simulink model "mVeh_tbm"  (R2020a)
settings: configuration reference "config_cnv" (kept outside this file)
undefined symbols (not defined in the file): Calib_pirelle_presSnr_x8, Calib_roadTriger_x6, Calib_tbm_brkBts_x8, Calib_tbm_ctr_x8, Calib_tbm_sensor_x4, Calib_tbm_strDistb_x8, Calib_tbm_supCtr_x8, CtrSet_tbm_enab_x8, FtIME_CAN_LINEoFF_ecuTbm_pd, Parm_tbmVeh_sig_max_numInvalid, Parm_tbmVeh_sig_tolerate_numInvalid, sigbuilder_block, SwCfg_cuTbm_simuCan
libraries: lib_canRx_msg_v2 x3, simulink x1, lib_decmp_Calib_tbm_brkPreTriger_x6 x1, lib_decmp_CtrSet_tbm_enab_x8 x1, libmf_bcu_spd_stsToValid x1, lib_decmp_Calib_tbm_sensor_x4 x1
settings Model: PauseTimes=30.8  Creator=jianjun.gao  LastModifiedBy=Administrator
settings ConfigSetRef: SourceName=config_cnv  SourceLocation=Base Workspace

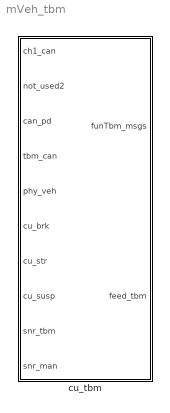
== system mVeh_tbm ==
  cu_tbm : Subsystem

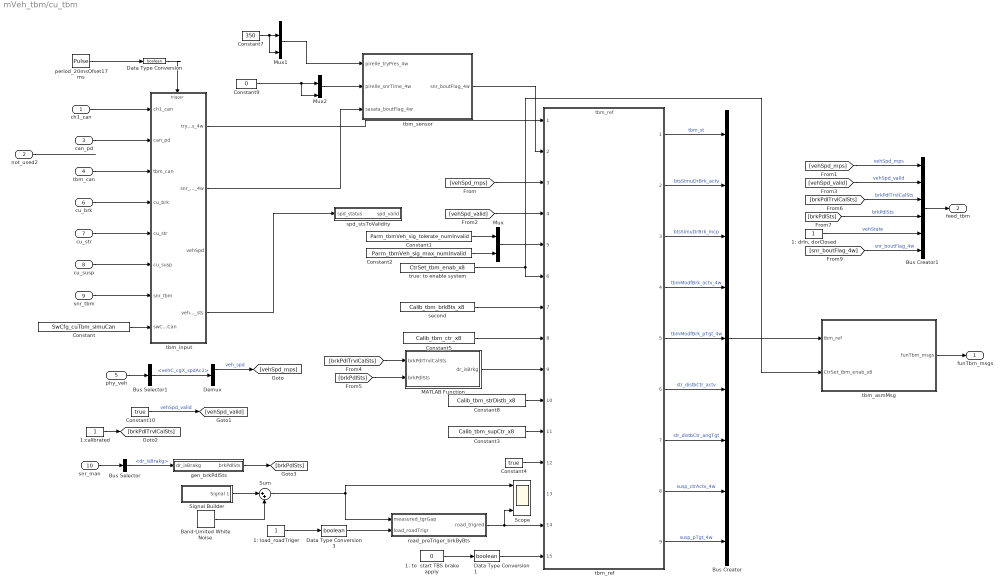
== system mVeh_tbm/cu_tbm ==
  ch1_can : Inport
  not_used2 : Inport  Port=2
  can_pd : Inport  Port=3
  tbm_can : Inport  Port=4
  phy_veh : Inport  Port=5
  cu_brk : Inport  Port=6
  cu_str : Inport  Port=7
  cu_susp : Inport  Port=8
  snr_tbm : Inport  Port=9
  snr_man : Inport  Port=10
  "1: drIn, dorClosed" : Constant  OutDataTypeStr=single  SampleTime=-1
  1: load_roadTriger : Constant  OutDataTypeStr=uint8  SampleTime=-1
  1: to  start TBS brake apply : Constant  Value=0  OutDataTypeStr=uint8  SampleTime=-1
  1:calibrated : Constant  OutDataTypeStr=uint8  SampleTime=-1
  Band-Limited White Noise : simulink/Sources/Band-Limited White Noise  Cov=[0.00000000001]  Ts=0.001  seed=[0]
  Bus Creator : BusCreator  Inputs=9
  Bus Creator1 : BusCreator  Inputs=6
  Bus Selector : BusSelector  OutputSignals=dr_isBrakg
  Bus Selector1 : BusSelector  OutputSignals=vehC_cgX_spdAc2
  Constant : Constant  Value=SwCfg_cuTbm_simuCan  OutDataTypeStr=boolean  SampleTime=-1
  Constant1 : Constant  Value=Parm_tbmVeh_sig_tolerate_numInvalid  OutDataTypeStr=int8  SampleTime=-1
  Constant10 : Constant  Value=true  OutDataTypeStr=boolean  SampleTime=-1
  Constant2 : Constant  Value=Parm_tbmVeh_sig_max_numInvalid  OutDataTypeStr=int8  SampleTime=-1
  Constant3 : Constant  Value=Calib_tbm_supCtr_x8  OutDataTypeStr=single  SampleTime=-1
  Constant4 : Constant  Value=true  OutDataTypeStr=boolean  SampleTime=-1
  Constant5 : Constant  Value=Calib_tbm_ctr_x8  OutDataTypeStr=single  SampleTime=-1
  Constant7 : Constant  Value=350  OutDataTypeStr=single  SampleTime=-1
  Constant8 : Constant  Value=Calib_tbm_strDistb_x8  OutDataTypeStr=single  SampleTime=-1
  Constant9 : Constant  Value=0  OutDataTypeStr=single  SampleTime=-1
  Data Type Conversion : DataTypeConversion  OutDataTypeStr=boolean  RndMeth=Nearest
  Data Type Conversion1 : DataTypeConversion  OutDataTypeStr=boolean  RndMeth=Nearest
  Data Type Conversion3 : DataTypeConversion  OutDataTypeStr=boolean  RndMeth=Nearest
  Demux : Demux  Outputs=2
  MATLAB Function : MATLAB Function  TreatAsAtomicUnit=on
  Mux : Mux  Inputs=2
  Mux1 : Mux
  Mux2 : Mux
  Scope : Scope  NumInputPorts=4
  Signal Builder : Subsystem  Tag=STV Subsys  LoadFcn=sigbuilder_block('load');  StartFcn=sigbuilder_block('start');  StopFcn=sigbuilder_block('stop');  ClipboardFcn=sigbuilder_block('clipboard');  mask(Sigbuilder block){tuvar=[0:10]}
      mask help: Simulink:masks:SigbuilderBlock_MD
      mask init:
      | if ~strcmp(get_param(bdroot(gcbh),'SimulationStatus'),'stopped') tuvar = sigbuilder_block('maskInit'); end
      settings: CopyFcn=sigbuilder_block('copy');  DeleteFcn=sigbuilder_block('delete');  ModelCloseFcn=sigbuilder_block('modelClose');  PreSaveFcn=sigbuilder_block('preSave');  PauseFcn=sigbuilder_block('pause');  ContinueFcn=sigbuilder_block('continue');  NameChangeFcn=sigbuilder_block('namechange');  OpenFcn=sigbuilder_block('open',[6 30 1428 680.25 ]);  CloseFcn=sigbuilder_block('close');
      mask Display: plot(0, 0, 100, 100,[2, 2, 32, 32, 2], [68, 8, 8, 68, 68],[32, 2], [38, 38], [32, 19, 2],[53, 60, 44], [32, 17, 17, 2],[16, 16, 31, 31]);txt = getActiveGroup(gcbh);text(2, 100, txt,'verticalAlignment', 'top');
  Sum : Sum  Inputs=|++
  gen_brkPdlSts : MATLAB Function  TreatAsAtomicUnit=on
  period_20msOfset17ms : DiscretePulseGenerator  PulseType=Time based  Period=0.02  PulseWidth=50  PhaseDelay=0.017
  road_preTriger_brkByBts : Subsystem
  second : Constant  Value=Calib_tbm_brkBts_x8  OutDataTypeStr=single  SampleTime=-1
  spd_stsToValidity : MATLAB Function  TreatAsAtomicUnit=on
  tbm_asmMsg : Subsystem
  tbm_input : Subsystem
  tbm_ref : ModelReference  ModelNameDialog=tbm_ref.slx  SimulationMode=Normal  ModelReferenceVersion=1.927
  tbm_sensor : Subsystem
  true: to enable system : Constant  Value=CtrSet_tbm_enab_x8  OutDataTypeStr=boolean  SampleTime=-1
  funTbm_msgs : Outport
  feed_tbm : Outport  Port=2
  wires:
  Mux2/1 -> tbm_sensor/2(pirelle_snrTime_4w)
  Constant9/1 -> Mux2/2, Mux2/4
  tbm_sensor/1(snr_boutFlag_4w) -> tbm_ref/2
  Mux1/1 -> tbm_sensor/1(pirelle_tryPres_4w)
  Constant7/1 -> Mux1/2, Mux1/4
  road_preTriger_brkByBts/1(road_trigred) -> tbm_ref/14, Scope/4
  Band-Limited White Noise/1 -> Sum/2
  Data Type Conversion3/1 -> road_preTriger_brkByBts/2(load_roadTrigr)
  1: load_roadTriger/1 -> Data Type Conversion3/1
  Signal Builder/1(Signal 1) -> Sum/1
  Sum/1 -> road_preTriger_brkByBts/1(measured_tgrGap), Scope/1
  [snr_boutFlag_4w] -> Bus Creator1/6  "snr_boutFlag_4w"
  "1: drIn, dorClosed"/1 -> Bus Creator1/5  "vehState"
  [brkPdlSts] -> Bus Creator1/4  "brkPdlSts"
  [brkPdlTrvlCalSts] -> Bus Creator1/3  "brkPdlTrvlCalSts"
  [brkPdlSts] -> MATLAB Function/2(brkPdlSts)
  MATLAB Function/1(dr_isBrkg) -> tbm_ref/9
  gen_brkPdlSts/1(brkPdlSts) -> [brkPdlSts]
  [brkPdlTrvlCalSts] -> MATLAB Function/1(brkPdlTrvlCalSts)
  1:calibrated/1 -> [brkPdlTrvlCalSts]
  [vehSpd_valid] -> Bus Creator1/2  "vehSpd_valid"
  [vehSpd_valid] -> tbm_ref/4
  Constant10/1 -> [vehSpd_valid]  "vehSpd_valid"
  [vehSpd_mps] -> Bus Creator1/1  "vehSpd_mps"
  [vehSpd_mps] -> tbm_ref/3
  Demux/1 -> [vehSpd_mps]  "veh_spd"
  Bus Creator1/1 -> feed_tbm/1
  Bus Selector1/1 -> Demux/1  "<vehC_cgX_spdAc2>"
  tbm_asmMsg/1(funTbm_msgs) -> funTbm_msgs/1
  tbm_ref/6 -> Bus Creator/6  "str_distbCtr_actv"
  tbm_ref/7 -> Bus Creator/7  "str_distbCtr_angTgt"
  Constant4/1 -> tbm_ref/12
  tbm_ref/9 -> Bus Creator/9  "susp_pTgt_4w"
  tbm_ref/8 -> Bus Creator/8  "susp_ctrActv_4w"
  Constant3/1 -> tbm_ref/11
  Constant8/1 -> tbm_ref/10
  tbm_ref/5 -> Bus Creator/5  "tbmModfBrk_pTgt_4w"
  tbm_ref/4 -> Bus Creator/4  "tbmModfBrk_actv_4w"
  Bus Selector/1 -> gen_brkPdlSts/1(dr_isBrakg)  "<dr_isBrakg>"
  Data Type Conversion1/1 -> tbm_ref/15
  second/1 -> tbm_ref/7
  snr_man/1 -> Bus Selector/1
  Bus Creator/1 -> tbm_asmMsg/1(tbm_ref)
  tbm_input/4(vehSpd_sts) -> spd_stsToValidity/1(spd_status)
  tbm_input/2(snr_boutFlag_4w) -> tbm_sensor/3(sasata_boutFlag_4w)
  tbm_input/1(tryPres_4w) -> tbm_ref/1
  Mux/1 -> tbm_ref/5
  1: to  start TBS brake apply/1 -> Data Type Conversion1/1
  true: to enable system/1 -> tbm_asmMsg/2(CtrSet_tbm_enab_x8), tbm_ref/6
  Constant5/1 -> tbm_ref/8
  Constant2/1 -> Mux/2
  Constant1/1 -> Mux/1
  Data Type Conversion/1 -> tbm_input/Trigger
  cu_brk/1 -> tbm_input/4(cu_brk)
  period_20msOfset17ms/1 -> Data Type Conversion/1
  Constant/1 -> tbm_input/8(swCfg_simuCan)
  tbm_ref/3 -> Bus Creator/3  "btsSimuDrBrk_mcp"
  tbm_ref/2 -> Bus Creator/2  "btsSimuDrBrk_actv"
  tbm_ref/1 -> Bus Creator/1  "tbm_st"
  tbm_can/1 -> tbm_input/3(tbm_can)
  can_pd/1 -> tbm_input/2(can_pd)
  not_used2/1 -> ?
  ch1_can/1 -> tbm_input/1(ch1_can)
  phy_veh/1 -> Bus Selector1/1
  cu_str/1 -> tbm_input/5(cu_str)
  cu_susp/1 -> tbm_input/6(cu_susp)
  snr_tbm/1 -> tbm_input/7(snr_tbm)

== system mVeh_tbm/cu_tbm/Signal Builder ==
  Demux : Demux  Tag=STV Demux  Outputs=1
      settings: DisplayOption=none
  FromWs : FromWorkspace  Tag=STV FromWs  VariableName=tuvar
      SigBuilderData=|
      | common.afterFinalStr = 'Extrapolate'
      | common.sampleTime = 0
      | dataSet.timeRange = [0 40]
      | dataSet.name = 'Group 1'
      | sbobj.Groups.Name = 'Group 1'
      | sbobj.Groups.Signals.Name = 'Signal 1'
      | sbobj.Groups.Signals.XData = [0 13 13 13.3 13.3 40]
      | sbobj.Groups.Signals.YData = [0.528 0.528 0.222 0.222 0.53 0.53]
      | sbobj.Groups.TimeRange = [0 40]
  Signal 1 : Outport  Tag=STV Outport
  wires:
  FromWs/1 -> Demux/1
  Demux/1 -> Signal 1/1

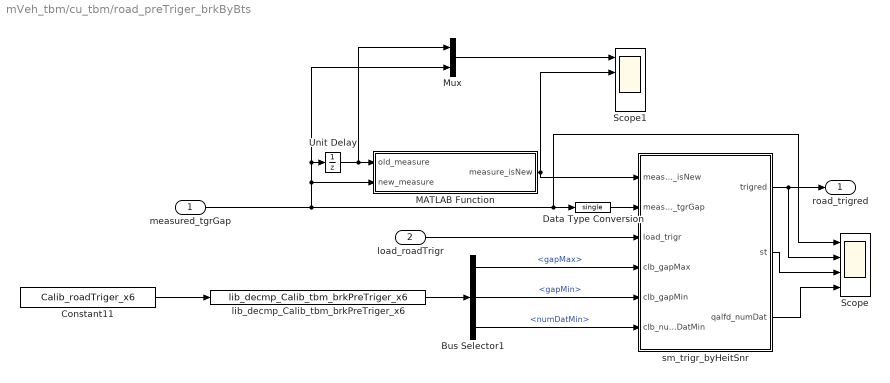
== system mVeh_tbm/cu_tbm/road_preTriger_brkByBts ==
  measured_tgrGap : Inport  OutDataTypeStr=double
  load_roadTrigr : Inport  Port=2  OutDataTypeStr=boolean
  Bus Selector1 : BusSelector  OutputSignals=gapMax,gapMin,numDatMin
  Constant11 : Constant  Value=Calib_roadTriger_x6  OutDataTypeStr=single  SampleTime=-1
  Data Type Conversion : DataTypeConversion  OutDataTypeStr=single
  MATLAB Function : MATLAB Function  TreatAsAtomicUnit=on
  Mux : Mux  Inputs=2
  Scope : Scope  NumInputPorts=4
  Scope1 : Scope  NumInputPorts=4
  Unit Delay : UnitDelay  SampleTime=-1  HasFrameUpgradeWarning=on
  lib_decmp_Calib_tbm_brkPreTriger_x6 : lib_decmp_Calib_tbm_brkPreTriger_x6/lib_decmp_Calib_tbm_brkPreTriger_x6  SystemSampleTime=-1  Latency=0  AutoFrameSizeCalculation=off
  sm_trigr_byHeitSnr : Stateflow chart  TreatAsAtomicUnit=on
  road_trigred : Outport
  wires:
  Data Type Conversion/1 -> sm_trigr_byHeitSnr/2(measured_tgrGap)
  Bus Selector1/3 -> sm_trigr_byHeitSnr/6(clb_numDatMin)  "<numDatMin>"
  Mux/1 -> Scope1/1
  sm_trigr_byHeitSnr/2(st) -> Scope/3
  sm_trigr_byHeitSnr/3(qalfd_numDat) -> Scope/4
  lib_decmp_Calib_tbm_brkPreTriger_x6/1 -> Bus Selector1/1
  Constant11/1 -> lib_decmp_Calib_tbm_brkPreTriger_x6/1
  sm_trigr_byHeitSnr/1(trigred) -> road_trigred/1, Scope/2
  load_roadTrigr/1 -> sm_trigr_byHeitSnr/3(load_trigr)
  measured_tgrGap/1 -> Data Type Conversion/1, Scope/1, MATLAB Function/2(new_measure), Unit Delay/1, Mux/2
  MATLAB Function/1(measure_isNew) -> Scope1/2, sm_trigr_byHeitSnr/1(measure_isNew)
  Unit Delay/1 -> MATLAB Function/1(old_measure), Mux/1
  Bus Selector1/1 -> sm_trigr_byHeitSnr/4(clb_gapMax)  "<gapMax>"
  Bus Selector1/2 -> sm_trigr_byHeitSnr/5(clb_gapMin)  "<gapMin>"

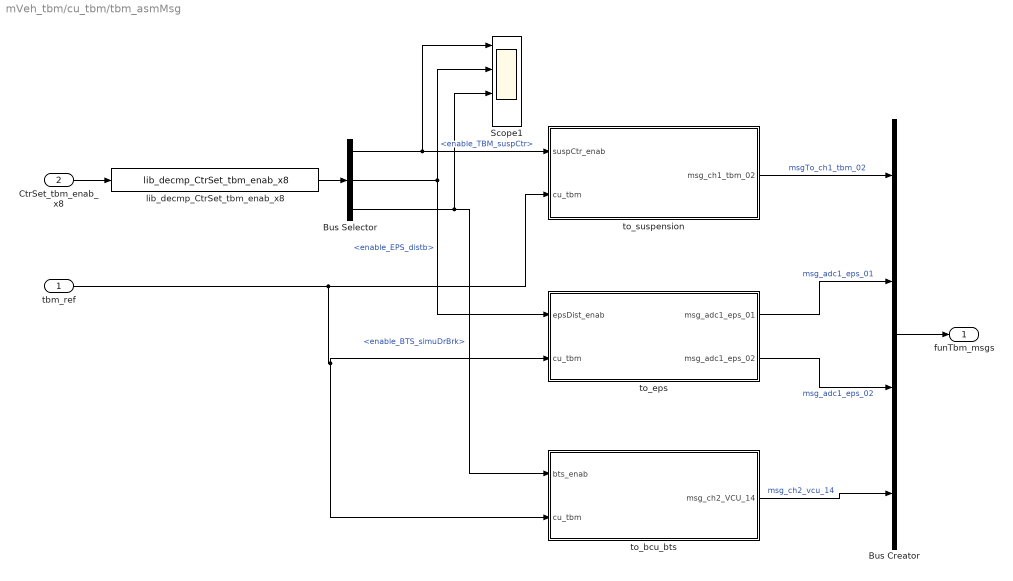
== system mVeh_tbm/cu_tbm/tbm_asmMsg ==
  tbm_ref : Inport
  CtrSet_tbm_enab_x8 : Inport  Port=2  OutDataTypeStr=boolean  PortDimensions=8
  Bus Creator : BusCreator  Inputs=4
  Bus Selector : BusSelector  OutputSignals=enable_TBM_suspCtr,enable_EPS_distb,enable_BTS_simuDrBrk
  Scope1 : Scope  NumInputPorts=4
  lib_decmp_CtrSet_tbm_enab_x8 : lib_decmp_CtrSet_tbm_enab_x8/lib_decmp_CtrSet_tbm_enab_x8  SystemSampleTime=-1  Latency=0  AutoFrameSizeCalculation=off
  to_bcu_bts : Subsystem
  to_eps : Subsystem
  to_suspension : Subsystem
  funTbm_msgs : Outport
  wires:
  Bus Creator/1 -> funTbm_msgs/1
  to_bcu_bts/1(msg_ch2_VCU_14) -> Bus Creator/4  "msg_ch2_vcu_14"
  to_eps/2(msg_adc1_eps_02) -> Bus Creator/3  "msg_adc1_eps_02"
  to_eps/1(msg_adc1_eps_01) -> Bus Creator/2  "msg_adc1_eps_01"
  to_suspension/1(msg_ch1_tbm_02) -> Bus Creator/1  "msgTo_ch1_tbm_02"
  Bus Selector/3 -> to_bcu_bts/1(bts_enab), Scope1/3  "<enable_BTS_simuDrBrk>"
  Bus Selector/2 -> to_eps/1(epsDist_enab), Scope1/2  "<enable_EPS_distb>"
  Bus Selector/1 -> to_suspension/1(suspCtr_enab), Scope1/1  "<enable_TBM_suspCtr>"
  lib_decmp_CtrSet_tbm_enab_x8/1 -> Bus Selector/1
  CtrSet_tbm_enab_x8/1 -> lib_decmp_CtrSet_tbm_enab_x8/1
  tbm_ref/1 -> to_suspension/2(cu_tbm), to_eps/2(cu_tbm), to_bcu_bts/2(cu_tbm)

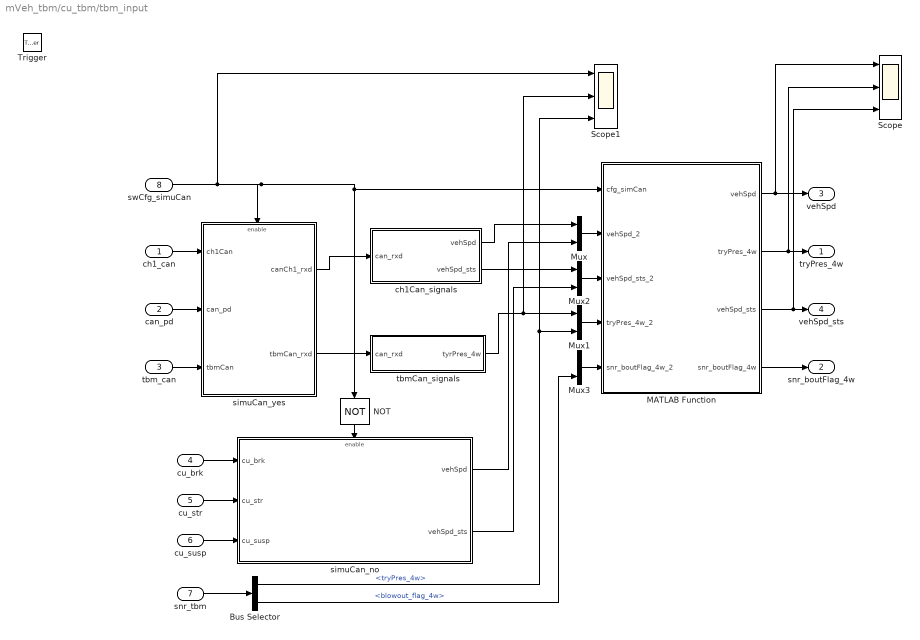
== system mVeh_tbm/cu_tbm/tbm_input ==
  ch1_can : Inport
  can_pd : Inport  Port=2
  tbm_can : Inport  Port=3
  cu_brk : Inport  Port=4
  cu_str : Inport  Port=5
  cu_susp : Inport  Port=6
  snr_tbm : Inport  Port=7
  swCfg_simuCan : Inport  Port=8
  Trigger : TriggerPort  TriggerType=either  VariantControl=Variant  PortDimensions=1
  Bus Selector : BusSelector  OutputSignals=tryPres_4w,blowout_flag_4w
  MATLAB Function : MATLAB Function  TreatAsAtomicUnit=on
  Mux{,1..3} (4 alike) : Mux  Inputs=2
  NOT : Logic  Operator=NOT  IconShape=distinctive  AllPortsSameDT=off  OutDataTypeStr=boolean
  Scope : Scope  NumInputPorts=3
  Scope1 : Scope  NumInputPorts=3
  ch1Can_signals : Subsystem
  simuCan_no : Subsystem
  simuCan_yes : Subsystem
  tbmCan_signals : Subsystem
  tryPres_4w : Outport
  snr_boutFlag_4w : Outport  Port=2
  vehSpd : Outport  Port=3
  vehSpd_sts : Outport  Port=4
  wires:
  MATLAB Function/4(snr_boutFlag_4w) -> snr_boutFlag_4w/1
  Mux3/1 -> MATLAB Function/5(snr_boutFlag_4w_2)
  Bus Selector/2 -> Mux3/2  "<blowout_flag_4w>"
  tbmCan_signals/1(tyrPres_4w) -> Mux1/1, Scope1/2
  simuCan_yes/2(tbmCan_rxd) -> tbmCan_signals/1(can_rxd)
  ch1Can_signals/2(vehSpd_sts) -> Mux2/1
  ch1Can_signals/1(vehSpd) -> Mux/1
  simuCan_yes/1(canCh1_rxd) -> ch1Can_signals/1(can_rxd)
  simuCan_no/2(vehSpd_sts) -> Mux2/2
  Mux2/1 -> MATLAB Function/3(vehSpd_sts_2)
  MATLAB Function/3(vehSpd_sts) -> Scope/3, vehSpd_sts/1
  MATLAB Function/2(tryPres_4w) -> Scope/2, tryPres_4w/1
  Mux1/1 -> MATLAB Function/4(tryPres_4w_2)
  MATLAB Function/1(vehSpd) -> Scope/1, vehSpd/1
  NOT/1 -> simuCan_no/Enable
  swCfg_simuCan/1 -> simuCan_yes/Enable, MATLAB Function/1(cfg_simCan), NOT/1, Scope1/1
  Mux/1 -> MATLAB Function/2(vehSpd_2)
  tbm_can/1 -> simuCan_yes/3(tbmCan)
  can_pd/1 -> simuCan_yes/2(can_pd)
  ch1_can/1 -> simuCan_yes/1(ch1Can)
  cu_susp/1 -> simuCan_no/3(cu_susp)
  cu_str/1 -> simuCan_no/2(cu_str)
  simuCan_no/1(vehSpd) -> Mux/2
  cu_brk/1 -> simuCan_no/1(cu_brk)
  snr_tbm/1 -> Bus Selector/1
  Bus Selector/1 -> Mux1/2, Scope1/3  "<tryPres_4w>"

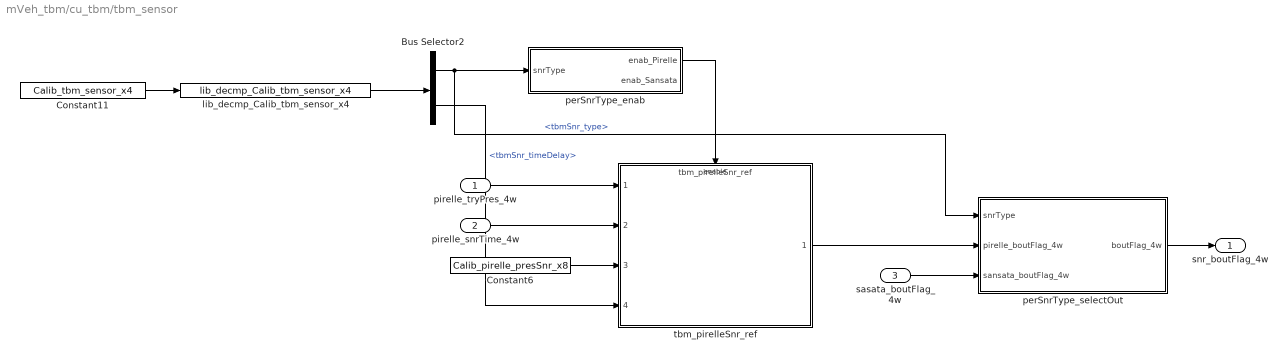
== system mVeh_tbm/cu_tbm/tbm_sensor ==
  pirelle_tryPres_4w : Inport  OutDataTypeStr=single  PortDimensions=4
  pirelle_snrTime_4w : Inport  Port=2  OutDataTypeStr=single  PortDimensions=4
  sasata_boutFlag_4w : Inport  Port=3  OutDataTypeStr=boolean  PortDimensions=4
  Bus Selector2 : BusSelector  OutputSignals=tbmSnr_type,tbmSnr_timeDelay
  Constant11 : Constant  Value=Calib_tbm_sensor_x4  SampleTime=-1
  Constant6 : Constant  Value=Calib_pirelle_presSnr_x8  OutDataTypeStr=single  SampleTime=-1
  lib_decmp_Calib_tbm_sensor_x4 : lib_decmp_Calib_tbm_sensor_x4/lib_decmp_Calib_tbm_sensor_x4  SystemSampleTime=-1  Latency=0  AutoFrameSizeCalculation=off
  perSnrType_enab : MATLAB Function  TreatAsAtomicUnit=on
  perSnrType_selectOut : MATLAB Function  TreatAsAtomicUnit=on
  tbm_pirelleSnr_ref : ModelReference  ModelNameDialog=tbm_pirelleSnr_ref.slx  SimulationMode=Normal  ModelReferenceVersion=1.851  EnablePortName=Enable  EnablePortStatesWhenEnabling=held
  snr_boutFlag_4w : Outport  OutDataTypeStr=boolean  PortDimensions=4
  wires:
  Bus Selector2/2 -> tbm_pirelleSnr_ref/4  "<tbmSnr_timeDelay>"
  pirelle_snrTime_4w/1 -> tbm_pirelleSnr_ref/2
  sasata_boutFlag_4w/1 -> perSnrType_selectOut/3(sansata_boutFlag_4w)
  tbm_pirelleSnr_ref/1 -> perSnrType_selectOut/2(pirelle_boutFlag_4w)
  perSnrType_selectOut/1(boutFlag_4w) -> snr_boutFlag_4w/1
  perSnrType_enab/1(enab_Pirelle) -> tbm_pirelleSnr_ref/Enable
  Bus Selector2/1 -> perSnrType_enab/1(snrType), perSnrType_selectOut/1(snrType)  "<tbmSnr_type>"
  Constant6/1 -> tbm_pirelleSnr_ref/3
  Constant11/1 -> lib_decmp_Calib_tbm_sensor_x4/1
  pirelle_tryPres_4w/1 -> tbm_pirelleSnr_ref/1
  lib_decmp_Calib_tbm_sensor_x4/1 -> Bus Selector2/1

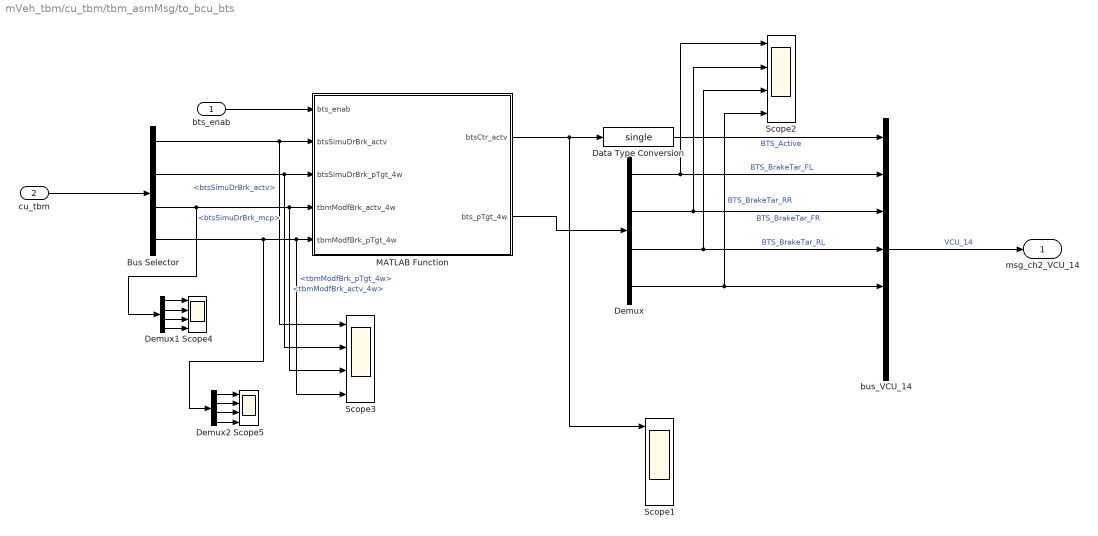
== system mVeh_tbm/cu_tbm/tbm_asmMsg/to_bcu_bts ==
  bts_enab : Inport
  cu_tbm : Inport  Port=2
  Bus Selector : BusSelector  OutputSignals=btsSimuDrBrk_actv,btsSimuDrBrk_mcp,tbmModfBrk_actv_4w,tbmModfBrk_pTgt_4w
  Data Type Conversion : DataTypeConversion  OutDataTypeStr=single  RndMeth=Nearest
  Demux : Demux
  Demux1 : Demux
  Demux2 : Demux
  MATLAB Function : MATLAB Function  TreatAsAtomicUnit=on
  Scope{1..5} (5 alike) : Scope  NumInputPorts=4
  bus_VCU_14 : BusCreator  Inputs=7
  msg_ch2_VCU_14 : Outport
  wires:
  Demux2/1 -> Scope5/1
  Demux2/2 -> Scope5/2
  Demux2/3 -> Scope5/3
  Demux2/4 -> Scope5/4
  Demux1/4 -> Scope4/4
  Demux1/3 -> Scope4/3
  Demux1/2 -> Scope4/2
  Demux1/1 -> Scope4/1
  MATLAB Function/2(bts_pTgt_4w) -> Demux/1
  Bus Selector/2 -> MATLAB Function/3(btsSimuDrBrk_pTgt_4w), Scope3/2  "<btsSimuDrBrk_mcp>"
  Bus Selector/4 -> MATLAB Function/5(tbmModfBrk_pTgt_4w), Scope3/4, Demux2/1  "<tbmModfBrk_pTgt_4w>"
  Bus Selector/3 -> MATLAB Function/4(tbmModfBrk_actv_4w), Scope3/3, Demux1/1  "<tbmModfBrk_actv_4w>"
  MATLAB Function/1(btsCtr_actv) -> Scope1/1, Data Type Conversion/1
  Bus Selector/1 -> MATLAB Function/2(btsSimuDrBrk_actv), Scope3/1  "<btsSimuDrBrk_actv>"
  Demux/4 -> bus_VCU_14/5, Scope2/4  "BTS_BrakeTar_RR"
  Demux/2 -> bus_VCU_14/3, Scope2/2  "BTS_BrakeTar_FR"
  bus_VCU_14/1 -> msg_ch2_VCU_14/1  "VCU_14"
  Data Type Conversion/1 -> bus_VCU_14/1  "BTS_Active"
  Demux/3 -> bus_VCU_14/4, Scope2/3  "BTS_BrakeTar_RL"
  Demux/1 -> bus_VCU_14/2, Scope2/1  "BTS_BrakeTar_FL"
  ? -> bus_VCU_14/7  "VCU_14_MsgCntr"
  ? -> bus_VCU_14/6  "VCU_14_CRC"
  cu_tbm/1 -> Bus Selector/1
  bts_enab/1 -> MATLAB Function/1(bts_enab)

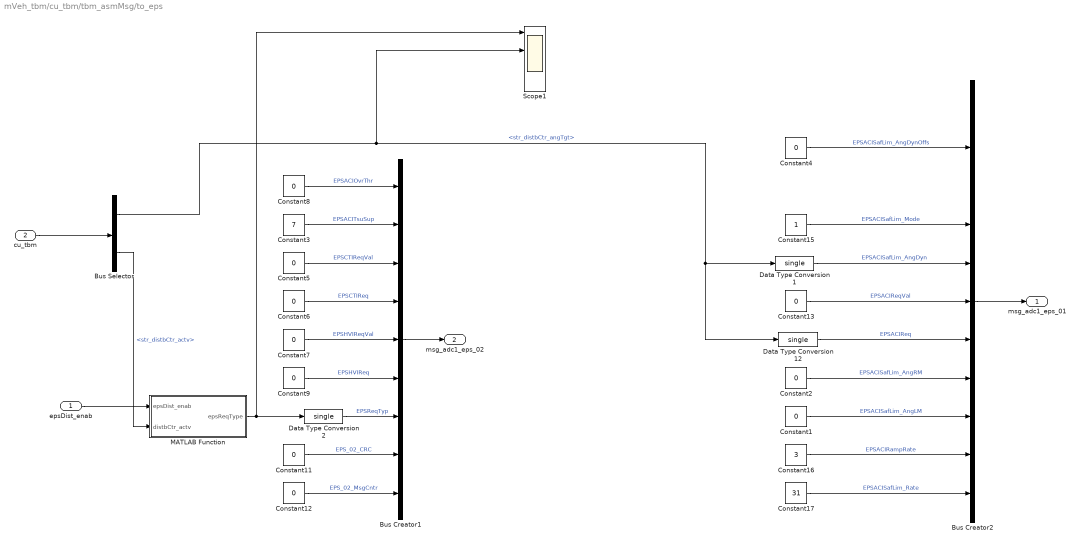
== system mVeh_tbm/cu_tbm/tbm_asmMsg/to_eps ==
  epsDist_enab : Inport
  cu_tbm : Inport  Port=2
  Bus Creator1 : BusCreator  Inputs=9
  Bus Creator2 : BusCreator  Inputs=11
  Bus Selector : BusSelector  OutputSignals=str_distbCtr_angTgt,str_distbCtr_actv
  Constant{1..2,4..9,11..13} (11 alike) : Constant  Value=0  OutDataTypeStr=single
  Constant15 : Constant  OutDataTypeStr=single
  Constant16 : Constant  Value=3  OutDataTypeStr=single
  Constant17 : Constant  Value=31  OutDataTypeStr=single
  Constant3 : Constant  Value=7  OutDataTypeStr=single
  Data Type Conversion1 : DataTypeConversion  OutDataTypeStr=single  RndMeth=Nearest
  Data Type Conversion12 : DataTypeConversion  OutDataTypeStr=single  RndMeth=Nearest
  Data Type Conversion2 : DataTypeConversion  OutDataTypeStr=single  RndMeth=Nearest
  MATLAB Function : MATLAB Function  TreatAsAtomicUnit=on
  Scope1 : Scope  NumInputPorts=4
  msg_adc1_eps_01 : Outport
  msg_adc1_eps_02 : Outport  Port=2
  wires:
  Data Type Conversion2/1 -> Bus Creator1/7  "EPSReqTyp"
  epsDist_enab/1 -> MATLAB Function/1(epsDist_enab)
  Bus Selector/2 -> MATLAB Function/2(distbCtr_actv)  "<str_distbCtr_actv>"
  cu_tbm/1 -> Bus Selector/1
  Constant15/1 -> Bus Creator2/4  "EPSACISafLim_Mode"
  Constant4/1 -> Bus Creator2/2  "EPSACISafLim_AngDynOffs"
  Constant5/1 -> Bus Creator1/3  "EPSCTIReqVal"
  Bus Creator1/1 -> msg_adc1_eps_02/1
  Constant8/1 -> Bus Creator1/1  "EPSACIOvrThr"
  Constant3/1 -> Bus Creator1/2  "EPSACITsuSup"
  Constant16/1 -> Bus Creator2/10  "EPSACIRampRate"
  Constant13/1 -> Bus Creator2/6  "EPSACIReqVal"
  Data Type Conversion12/1 -> Bus Creator2/7  "EPSACIReq"
  Constant6/1 -> Bus Creator1/4  "EPSCTIReq"
  Constant7/1 -> Bus Creator1/5  "EPSHVIReqVal"
  Bus Creator2/1 -> msg_adc1_eps_01/1
  Constant1/1 -> Bus Creator2/9  "EPSACISafLim_AngLM"
  Constant12/1 -> Bus Creator1/9  "EPS_02_MsgCntr"
  Data Type Conversion1/1 -> Bus Creator2/5  "EPSACISafLim_AngDyn"
  Constant17/1 -> Bus Creator2/11  "EPSACISafLim_Rate"
  MATLAB Function/1(epsReqType) -> Data Type Conversion2/1, Scope1/1
  Constant2/1 -> Bus Creator2/8  "EPSACISafLim_AngRM"
  ? -> Bus Creator2/1  "EPS_01_CRC"
  Constant11/1 -> Bus Creator1/8  "EPS_02_CRC"
  Constant9/1 -> Bus Creator1/6  "EPSHVIReq"
  Bus Selector/1 -> Data Type Conversion1/1, Data Type Conversion12/1, Scope1/2  "<str_distbCtr_angTgt>"
  ? -> Bus Creator2/3  "EPS_01_MsgCntr"

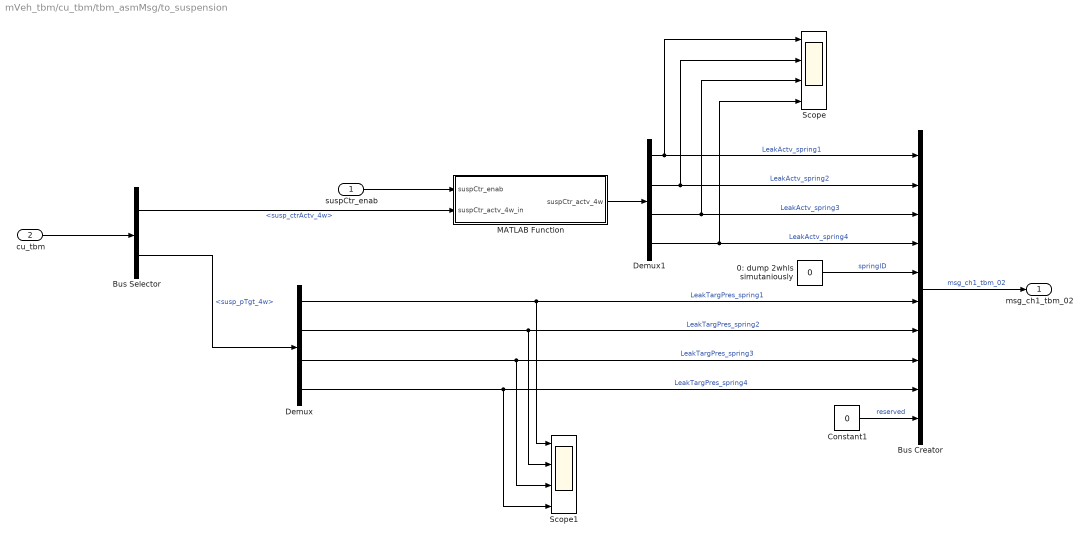
== system mVeh_tbm/cu_tbm/tbm_asmMsg/to_suspension ==
  suspCtr_enab : Inport
  cu_tbm : Inport  Port=2
  0: dump 2whls simutaniously : Constant  Value=0  OutDataTypeStr=single
  Bus Creator : BusCreator  Inputs=10
  Bus Selector : BusSelector  OutputSignals=susp_ctrActv_4w,susp_pTgt_4w
  Constant1 : Constant  Value=0  OutDataTypeStr=single
  Demux : Demux
  Demux1 : Demux
  MATLAB Function : MATLAB Function  TreatAsAtomicUnit=on
  Scope : Scope  NumInputPorts=4
  Scope1 : Scope  NumInputPorts=4
  msg_ch1_tbm_02 : Outport
  wires:
  suspCtr_enab/1 -> MATLAB Function/1(suspCtr_enab)
  MATLAB Function/1(suspCtr_actv_4w) -> Demux1/1
  Bus Selector/1 -> MATLAB Function/2(suspCtr_actv_4w_in)  "<susp_ctrActv_4w>"
  Bus Selector/2 -> Demux/1  "<susp_pTgt_4w>"
  Bus Creator/1 -> msg_ch1_tbm_02/1  "msg_ch1_tbm_02"
  Demux/1 -> Bus Creator/6, Scope1/1  "LeakTargPres_spring1"
  Demux1/3 -> Bus Creator/3, Scope/3  "LeakActv_spring3"
  Demux1/2 -> Bus Creator/2, Scope/2  "LeakActv_spring2"
  Constant1/1 -> Bus Creator/10  "reserved"
  Demux1/1 -> Bus Creator/1, Scope/1  "LeakActv_spring1"
  Demux/4 -> Bus Creator/9, Scope1/4  "LeakTargPres_spring4"
  Demux/3 -> Bus Creator/8, Scope1/3  "LeakTargPres_spring3"
  Demux/2 -> Bus Creator/7, Scope1/2  "LeakTargPres_spring2"
  Demux1/4 -> Bus Creator/4, Scope/4  "LeakActv_spring4"
  0: dump 2whls simutaniously/1 -> Bus Creator/5  "springID"
  cu_tbm/1 -> Bus Selector/1

== system mVeh_tbm/cu_tbm/tbm_input/ch1Can_signals ==
  can_rxd : Inport
  Bus Selector1 : BusSelector  OutputSignals=BCU_04_rxd
  Bus Selector2 : BusSelector  OutputSignals=BCU_04.VehSpd,BCU_04.VehSpdSts
  vehSpd : Outport
  vehSpd_sts : Outport  Port=2
  wires:
  Bus Selector2/2 -> vehSpd_sts/1  "<VehSpdSts>"
  Bus Selector2/1 -> vehSpd/1  "<VehSpd>"
  Bus Selector1/1 -> Bus Selector2/1  "<BCU_04_rxd>"
  can_rxd/1 -> Bus Selector1/1

== system mVeh_tbm/cu_tbm/tbm_input/simuCan_no ==
  cu_brk : Inport
  cu_str : Inport  Port=2
  cu_susp : Inport  Port=3
  Enable : EnablePort
  Bus Selector1 : BusSelector  OutputSignals=vehSpd,vehSpd_valid
  libmf_spd_validToSts : libmf_bcu_spd_stsToValid/libmf_spd_validToSts  SystemSampleTime=-1  Latency=0  AutoFrameSizeCalculation=off
  vehSpd : Outport
  vehSpd_sts : Outport  Port=2
  wires:
  libmf_spd_validToSts/1 -> vehSpd_sts/1
  Bus Selector1/2 -> libmf_spd_validToSts/1  "<vehSpd_valid>"
  cu_brk/1 -> Bus Selector1/1
  Bus Selector1/1 -> vehSpd/1  "<vehSpd>"

== system mVeh_tbm/cu_tbm/tbm_input/simuCan_yes ==
  ch1Can : Inport
  can_pd : Inport  Port=2
  tbmCan : Inport  Port=3
  Enable : EnablePort
  ch1Can_rx : Subsystem
  tbmCan_rx : Subsystem
  canCh1_rxd : Outport
  tbmCan_rxd : Outport  Port=2
  wires:
  tbmCan_rx/1(can_rxd) -> tbmCan_rxd/1
  tbmCan/1 -> tbmCan_rx/1(can)
  ch1Can_rx/1(can_rxd) -> canCh1_rxd/1
  ch1Can/1 -> ch1Can_rx/1(can)

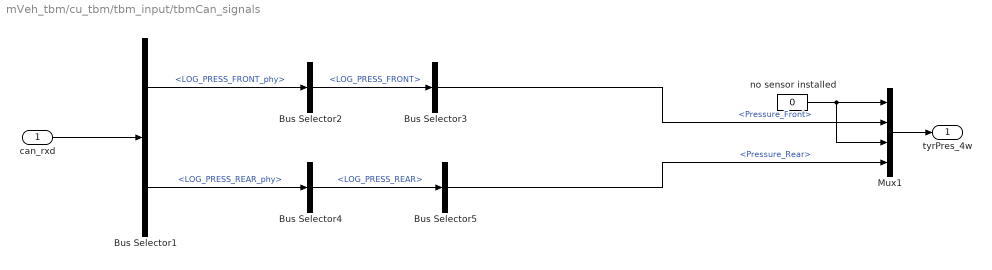
== system mVeh_tbm/cu_tbm/tbm_input/tbmCan_signals ==
  can_rxd : Inport
  Bus Selector1 : BusSelector  OutputSignals=LOG_PRESS_FRONT_phy,LOG_PRESS_REAR_phy
  Bus Selector2 : BusSelector  OutputSignals=LOG_PRESS_FRONT
  Bus Selector3 : BusSelector  OutputSignals=Pressure_Front
  Bus Selector4 : BusSelector  OutputSignals=LOG_PRESS_REAR
  Bus Selector5 : BusSelector  OutputSignals=Pressure_Rear
  Mux1 : Mux
  no sensor installed : Constant  Value=0  OutDataTypeStr=single  SampleTime=-1
  tyrPres_4w : Outport
  wires:
  no sensor installed/1 -> Mux1/1, Mux1/3
  Mux1/1 -> tyrPres_4w/1
  Bus Selector4/1 -> Bus Selector5/1  "<LOG_PRESS_REAR>"
  Bus Selector5/1 -> Mux1/4  "<Pressure_Rear>"
  Bus Selector3/1 -> Mux1/2  "<Pressure_Front>"
  Bus Selector1/2 -> Bus Selector4/1  "<LOG_PRESS_REAR_phy>"
  can_rxd/1 -> Bus Selector1/1
  Bus Selector1/1 -> Bus Selector2/1  "<LOG_PRESS_FRONT_phy>"
  Bus Selector2/1 -> Bus Selector3/1  "<LOG_PRESS_FRONT>"

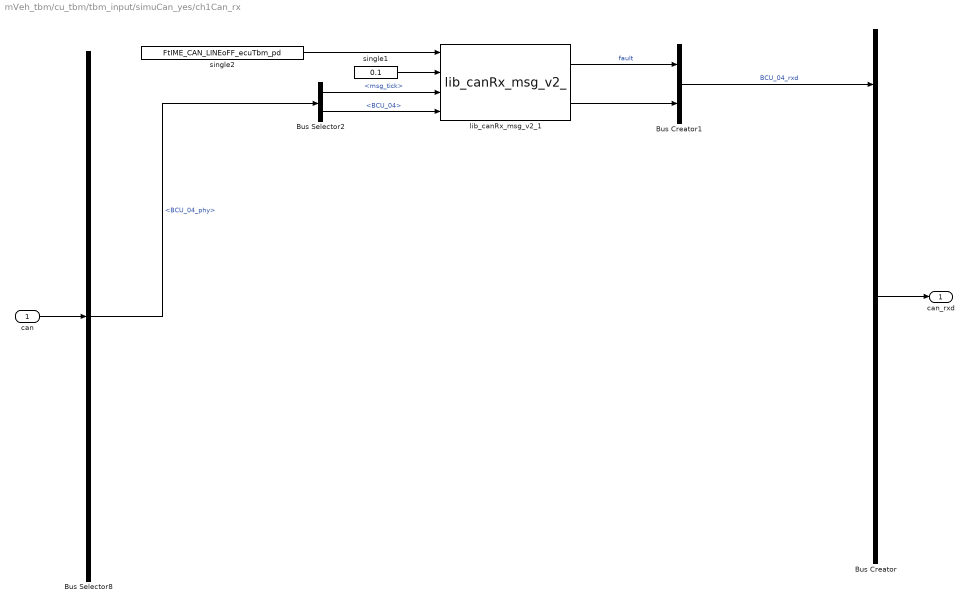
== system mVeh_tbm/cu_tbm/tbm_input/simuCan_yes/ch1Can_rx ==
  can : Inport
  Bus Creator : BusCreator  Inputs=5
  Bus Creator1 : BusCreator  Inputs=2
  Bus Selector2 : BusSelector  OutputSignals=msg_tick,BCU_04
  Bus Selector8 : BusSelector  OutputSignals=bcu.BCU_04_phy
  lib_canRx_msg_v2_1 : lib_canRx_msg_v2/lib_canRx_msg_v2_  SystemSampleTime=-1  Latency=0  AutoFrameSizeCalculation=off
  single1 : Constant  Value=0.1  OutDataTypeStr=single
  single2 : Constant  Value=FtIME_CAN_LINEoFF_ecuTbm_pd  OutDataTypeStr=single
  can_rxd : Outport  VectorParamsAs1DForOutWhenUnconnected=off
  wires:
  Bus Selector2/2 -> lib_canRx_msg_v2_1/4  "<BCU_04>"
  lib_canRx_msg_v2_1/1 -> Bus Creator1/1  "fault"
  Bus Selector2/1 -> lib_canRx_msg_v2_1/3  "<msg_tick>"
  single1/1 -> lib_canRx_msg_v2_1/2
  lib_canRx_msg_v2_1/2 -> Bus Creator1/2
  Bus Creator1/1 -> Bus Creator/1  "BCU_04_rxd"
  single2/1 -> lib_canRx_msg_v2_1/1
  can/1 -> Bus Selector8/1
  Bus Selector8/1 -> Bus Selector2/1  "<BCU_04_phy>"
  Bus Creator/1 -> can_rxd/1

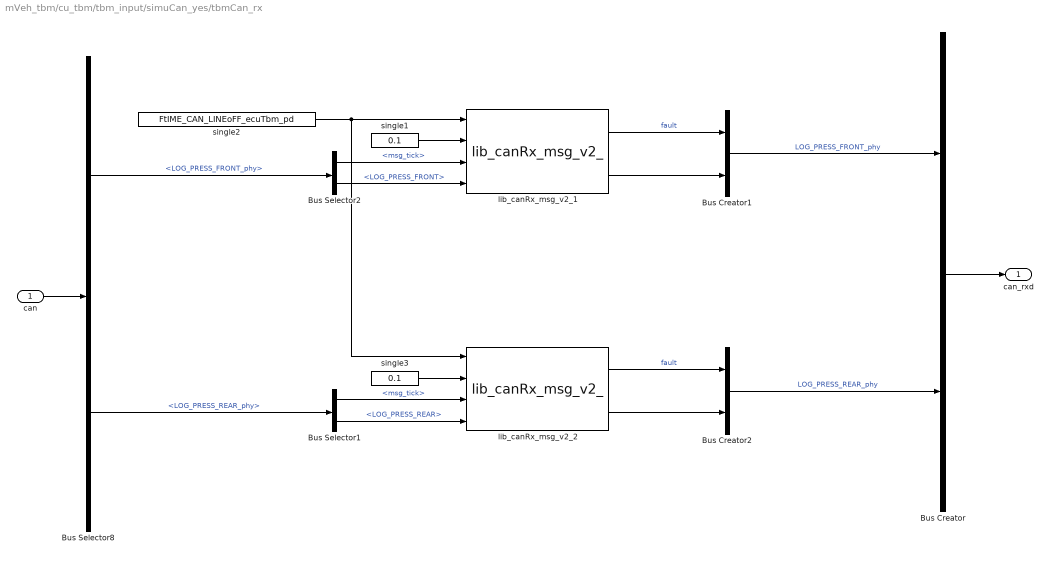
== system mVeh_tbm/cu_tbm/tbm_input/simuCan_yes/tbmCan_rx ==
  can : Inport
  Bus Creator : BusCreator  Inputs=2
  Bus Creator1 : BusCreator  Inputs=2
  Bus Creator2 : BusCreator  Inputs=2
  Bus Selector1 : BusSelector  OutputSignals=msg_tick,LOG_PRESS_REAR
  Bus Selector2 : BusSelector  OutputSignals=msg_tick,LOG_PRESS_FRONT
  Bus Selector8 : BusSelector  OutputSignals=tbm_pSnr.LOG_PRESS_FRONT_phy,tbm_pSnr.LOG_PRESS_REAR_phy
  lib_canRx_msg_v2_1 : lib_canRx_msg_v2/lib_canRx_msg_v2_  SystemSampleTime=-1  Latency=0  AutoFrameSizeCalculation=off
  lib_canRx_msg_v2_2 : lib_canRx_msg_v2/lib_canRx_msg_v2_  SystemSampleTime=-1  Latency=0  AutoFrameSizeCalculation=off
  single1 : Constant  Value=0.1  OutDataTypeStr=single
  single2 : Constant  Value=FtIME_CAN_LINEoFF_ecuTbm_pd  OutDataTypeStr=single
  single3 : Constant  Value=0.1  OutDataTypeStr=single
  can_rxd : Outport  VectorParamsAs1DForOutWhenUnconnected=off
  wires:
  Bus Selector8/2 -> Bus Selector1/1  "<LOG_PRESS_REAR_phy>"
  lib_canRx_msg_v2_2/1 -> Bus Creator2/1  "fault"
  lib_canRx_msg_v2_2/2 -> Bus Creator2/2
  single2/1 -> lib_canRx_msg_v2_1/1, lib_canRx_msg_v2_2/1
  Bus Selector1/2 -> lib_canRx_msg_v2_2/4  "<LOG_PRESS_REAR>"
  Bus Creator2/1 -> Bus Creator/2  "LOG_PRESS_REAR_phy"
  single3/1 -> lib_canRx_msg_v2_2/2
  Bus Selector1/1 -> lib_canRx_msg_v2_2/3  "<msg_tick>"
  Bus Creator/1 -> can_rxd/1
  Bus Selector8/1 -> Bus Selector2/1  "<LOG_PRESS_FRONT_phy>"
  can/1 -> Bus Selector8/1
  Bus Creator1/1 -> Bus Creator/1  "LOG_PRESS_FRONT_phy"
  lib_canRx_msg_v2_1/2 -> Bus Creator1/2
  single1/1 -> lib_canRx_msg_v2_1/2
  Bus Selector2/1 -> lib_canRx_msg_v2_1/3  "<msg_tick>"
  lib_canRx_msg_v2_1/1 -> Bus Creator1/1  "fault"
  Bus Selector2/2 -> lib_canRx_msg_v2_1/4  "<LOG_PRESS_FRONT>"

== matlab function mVeh_tbm/cu_tbm/road_preTriger_brkByBts/MATLAB Function ==
  data: old_measure input double; measure_isNew output boolean; new_measure input double
function measure_isNew = fcn(old_measure, new_measure)

measure_isNew = false;

if old_measure ~= new_measure
    measure_isNew = true;
end

== stateflow chart mVeh_tbm/cu_tbm/road_preTriger_brkByBts/sm_trigr_byHeitSnr ==
  state trigred
    en:
    st = 3;    trigred = true;
  state disregard
    en:
    st = 0;    trigred = false;
  state trigring
    en:
    st = 2;    trigred = false;
    state qualifed
      en:
      qalfd_numDat = qalfd_numDat +1;
    state unqualifed
      en:
      qalfd_numDat = qalfd_numDat -1;
    qualifed -> (junction 32)
    (junction 19) -> qualifed [order 1] : [      (measured_tgrGap < clb_gapMax) ...
        |   && (measured_tgrGap > clb_gapMin) ]
    (junction 32) -> (junction 19) : [measure_isNew]
    unqualifed -> (junction 32)
    (junction 19) -> unqualifed [order 2]
  state watch_for_trigr
    en:
    st = 1;    trigred = false;    qalfd_numDat = 0;
  (default) -> disregard
  trigred -> disregard : after(5, sec)
  trigring -> trigred [order 1] : [qalfd_numDat > clb_numDatMin ]
  disregard -> watch_for_trigr : [ load_trigr ]
  watch_for_trigr -> disregard [order 2] : [ ~load_trigr ]
  watch_for_trigr -> (junction 32) [order 1]
  trigring -> watch_for_trigr [order 2] : [qalfd_numDat <= 0 ]
  data: measure_isNew input boolean; measured_tgrGap input single size=1; load_trigr input boolean; clb_gapMax input single size=1; clb_gapMin input single size=1; trigred output boolean; clb_numDatMin input uint8 size=1; st output uint8; qalfd_numDat output uint8 size=1

== matlab function mVeh_tbm/cu_tbm/tbm_sensor/perSnrType_enab ==
  data: snrType input Enum: Enum_tbm_snrType; enab_Pirelle output boolean; enab_Sansata output boolean
function [enab_Pirelle,enab_Sansata] = fcn(snrType)

enab_Pirelle = false;
enab_Sansata = false;

switch snrType
    case Enum_tbm_snrType.Pirelle
        enab_Pirelle = true;
    case Enum_tbm_snrType.Sansata  
        enab_Sansata = true;
    
end

== matlab function mVeh_tbm/cu_tbm/tbm_sensor/perSnrType_selectOut ==
  data: snrType input Enum: Enum_tbm_snrType; boutFlag_4w output boolean size=4; pirelle_boutFlag_4w input boolean size=4; sansata_boutFlag_4w input boolean size=4
function boutFlag_4w  = fcn(snrType, pirelle_boutFlag_4w, sansata_boutFlag_4w)

boutFlag_4w = [false; false; false; false];

switch snrType
    case Enum_tbm_snrType.Pirelle
        boutFlag_4w = pirelle_boutFlag_4w;
    case Enum_tbm_snrType.Sansata  
        boutFlag_4w = sansata_boutFlag_4w;
    
end

== matlab function mVeh_tbm/cu_tbm/tbm_input/MATLAB Function ==
  data: cfg_simCan input boolean; vehSpd output single; vehSpd_2 input single; tryPres_4w output single size=4; vehSpd_sts output uint8; vehSpd_sts_2 input uint8; tryPres_4w_2 input single size=8; snr_boutFlag_4w_2 input boolean size=8; snr_boutFlag_4w output boolean size=4
function [vehSpd,tryPres_4w, vehSpd_sts, snr_boutFlag_4w] = fcn(cfg_simCan, vehSpd_2, vehSpd_sts_2, tryPres_4w_2, snr_boutFlag_4w_2)

if cfg_simCan
    i = uint8(1);
else
    i = uint8(2); 
end

vehSpd          = vehSpd_2(i);
vehSpd_sts    = vehSpd_sts_2(i);

if cfg_simCan
    tryPres_4w = tryPres_4w_2(1:4);
    snr_boutFlag_4w = snr_boutFlag_4w_2(1:4);
else
    tryPres_4w = tryPres_4w_2(5:8);
    snr_boutFlag_4w = snr_boutFlag_4w_2(5:8);
end

== matlab function mVeh_tbm/cu_tbm/tbm_asmMsg/to_suspension/MATLAB Function ==
  data: suspCtr_enab input boolean; suspCtr_actv_4w output boolean size=4; suspCtr_actv_4w_in input boolean size=4
function suspCtr_actv_4w = fcn(suspCtr_enab, suspCtr_actv_4w_in)

suspCtr_actv_4w = [false; false; false; false];

if suspCtr_enab
  suspCtr_actv_4w = suspCtr_actv_4w_in;  
    
end

== matlab function mVeh_tbm/cu_tbm/gen_brkPdlSts ==
  data: dr_isBrakg input boolean; brkPdlSts output uint8
function brkPdlSts = fcn(dr_isBrakg)

brkPdlSts = uint8(0);

if dr_isBrakg
    brkPdlSts = uint8(1);
end

== matlab function mVeh_tbm/cu_tbm/tbm_asmMsg/to_bcu_bts/MATLAB Function ==
  data: btsCtr_actv output boolean; bts_enab input boolean; btsSimuDrBrk_actv input boolean; btsSimuDrBrk_pTgt_4w input single; bts_pTgt_4w output single size=4; tbmModfBrk_actv_4w input boolean size=4; tbmModfBrk_pTgt_4w input single size=4
function [btsCtr_actv, bts_pTgt_4w] = fcn (bts_enab, btsSimuDrBrk_actv, btsSimuDrBrk_pTgt_4w, tbmModfBrk_actv_4w, tbmModfBrk_pTgt_4w)

btsCtr_actv = false;
bts_pTgt_4w = [single(0); single(0); single(0); single(0)];

if bts_enab && btsSimuDrBrk_actv
    pTgt_4w = btsSimuDrBrk_pTgt_4w;
    btsCtr_actv = true;
    
    for w = 1:4
       if  tbmModfBrk_actv_4w(w) 
           pTgt_4w(w) = tbmModfBrk_pTgt_4w (w);
           
       end        
    end 
    bts_pTgt_4w = pTgt_4w; 
    
end

== matlab function mVeh_tbm/cu_tbm/spd_stsToValidity ==
  data: spd_valid output boolean; spd_status input uint8
function spd_valid  = fcn(spd_status)

if spd_status == 0 
    spd_valid = true; 
else
    spd_valid = false; 
end

== matlab function mVeh_tbm/cu_tbm/MATLAB Function ==
  data: brkPdlTrvlCalSts input uint8; dr_isBrkg output boolean; brkPdlSts input uint8
function dr_isBrkg = fcn(brkPdlTrvlCalSts, brkPdlSts)


dr_isBrkg = false; 

if    ( brkPdlTrvlCalSts == uint8(1) ) ...      % 1 is brake pedal sensor calibrated
   && ( brkPdlSts == uint8(1)  )                % 1 is brkPdl pressed  

    dr_isBrkg = true; 


end

== matlab function mVeh_tbm/cu_tbm/tbm_asmMsg/to_eps/MATLAB Function ==
  data: epsDist_enab input boolean; distbCtr_actv input boolean; epsReqType output uint8
function epsReqType = fcn (epsDist_enab, distbCtr_actv)

epsReqType = uint8(0);

if epsDist_enab && distbCtr_actv
    epsReqType = uint8(1);
end
